simulink model "ES011A_DualEcuIdn"  (R2013b)
settings: Solver=FixedStepDiscrete  SolverMode=SingleTasking  StartTime=0.0  StopTime=1  FixedStep=0.002  RelTol=1e-3
values from neighbouring files (symbols this model uses):
  ECUCOMTIOUTFLT_CNT_U08 = DataDict.Constant    [ES011A_DualEcuIdn_DataDict.m]
  ECUID1_CNT_U08 = DataDict.Constant    [ES011A_DualEcuIdn_DataDict.m]
  ECUID2_CNT_U08 = DataDict.Constant    [ES011A_DualEcuIdn_DataDict.m]
  ECUIDINVLD_CNT_U08 = DataDict.Constant    [ES011A_DualEcuIdn_DataDict.m]
  IDENTCLECUIDNFLT_CNT_U08 = DataDict.Constant    [ES011A_DualEcuIdn_DataDict.m]
  IMCARBN_DUALECUIDNSECDRYECUIDN_CNT_U16 = DataDict.Constant    [ES011A_DualEcuIdn_DataDict.m]
  PRIMECUIDNOTREADFLT_CNT_U08 = DataDict.Constant    [ES011A_DualEcuIdn_DataDict.m]
  PRIMECUINVLDIDFLT_CNT_U08 = DataDict.Constant    [ES011A_DualEcuIdn_DataDict.m]
  SECDRYECUIDNOTREADFLT_CNT_U08 = DataDict.Constant    [ES011A_DualEcuIdn_DataDict.m]
  SECDRYECUIDNREQTIOUTVAL_CNT_U08 = DataDict.Constant    [ES011A_DualEcuIdn_DataDict.m]
  SECDRYECUINVLDIDFLT_CNT_U08 = DataDict.Constant    [ES011A_DualEcuIdn_DataDict.m]
  SECDRYECUREQIDTIOUTFLT_CNT_U08 = DataDict.Constant    [ES011A_DualEcuIdn_DataDict.m]
  VLDECUID_CNT_U08 = DataDict.Constant    [ES011A_DualEcuIdn_DataDict.m]
undefined symbols (not defined in the file or in its folder): NtcNr1, NtcSts1, sigbuilder_block
libraries: simulink x2
(part 2 of 2)

== system ES011A_DualEcuIdn/DualEcuIdn/DualEcuIdnPer1/Evaluation Not Complete/Set Diagnostic 0x0B9/Pass NTC/CopyRight2 ==

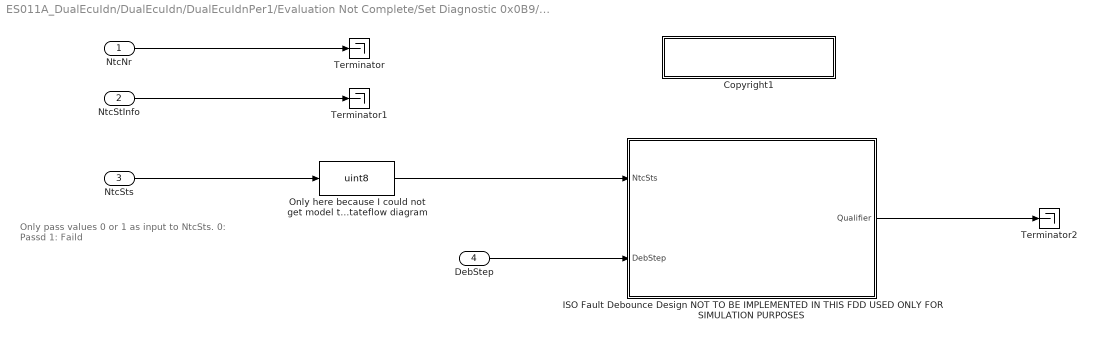
== system ES011A_DualEcuIdn/DualEcuIdn/DualEcuIdnPer1/Evaluation Not Complete/Set Diagnostic 0x0B9/Pass NTC/SetNtcSts ==
  note: Only pass values 0 or 1 as input to NtcSts.
      | 0: Passd
      | 1: Faild
  NtcNr : Inport
  NtcStInfo : Inport  Port=2
  NtcSts : Inport  Port=3  OutDataTypeStr=uint8
  DebStep : Inport  Port=4  OutDataTypeStr=uint16
  Copyright1 : Subsystem  Description=|  mask(Copyright Information){none=on}
      | Copyright info block.                                               
      |                                                                     
      | Place copyright information at the top of every subsystem in design.
      mask prompts: none "No parameters"
      mask help: Place copyright information at the top of every subsystem in design.
      mask Display:
      | NxtrConf = 'Nexteer Confidential';
      | 
      | sys = bdroot; %handle for the current model ("system")
      | first = get_param(sys,'Created');
      | if(isempty(first))
      |     first = datestr(now,'yyyy');
      | else
      |     first = first(end-3:end);  %year is last four digits
      | end
      | 
      | last = get_param(sys,'LastModifiedDate');
      | if isempty(last)
      |     last = datestr(now,'yyyy');
      | else
      |     last = last(end-3:end);
      | end
      | 
      | if strcmp(first,last)
      |     fprintf('%s\nCopyright  %s Nexteer',NxtrConf,first);
      | else
      |     fprintf('%s\n%s%s-%s Nexteer',NxtrConf,char(169),first,last);
      | end
  ISO Fault Debounce Design NOT TO BE IMPLEMENTED IN THIS FDD USED ONLY FOR SIMULATION PURPOSES : Stateflow chart  TreatAsAtomicUnit=on
  Only here because I could not get model to run with enumerations in the stateflow diagram : DataTypeConversion  OutDataTypeStr=uint8
  Terminator : Terminator
  Terminator1 : Terminator
  Terminator2 : Terminator
  wires:
  NtcStInfo/1 -> Terminator1/1
  NtcNr/1 -> Terminator/1
  NtcSts/1 -> Only here because I could not get model to run with enumerations in the stateflow diagram/1
  DebStep/1 -> ISO Fault Debounce Design NOT TO BE IMPLEMENTED IN THIS FDD USED ONLY FOR SIMULATION PURPOSES/2(DebStep)
  ISO Fault Debounce Design NOT TO BE IMPLEMENTED IN THIS FDD USED ONLY FOR SIMULATION PURPOSES/1(Qualifier) -> Terminator2/1
  Only here because I could not get model to run with enumerations in the stateflow diagram/1 -> ISO Fault Debounce Design NOT TO BE IMPLEMENTED IN THIS FDD USED ONLY FOR SIMULATION PURPOSES/1(NtcSts)

== system ES011A_DualEcuIdn/DualEcuIdn/DualEcuIdnPer1/Evaluation Not Complete/Valid Data and E_OK/Different ECU Id/All Good ==
  Action Port : ActionPort  ActionType=else
  CopyRight2 : Subsystem  Description=|  mask(Copyright Information){none=on}
      | Copyright info block.                                               
      |                                                                     
      | Place copyright information at the top of every subsystem in design.
      mask prompts: none "No parameters"
      mask help: Place copyright information at the top of every subsystem in design.
      mask Display:
      | NxtrConf = 'Nexteer Confidential';
      | 
      | sys = bdroot; %handle for the current model ("system")
      | first = get_param(sys,'Created');
      | first = first(end-3:end);  %year is last four digits
      | 
      | last = get_param(sys,'LastModifiedDate');
      | if isempty(last)
      |     last = datestr(now,'yyyy');
      | else
      |     last = last(end-3:end);
      | end
      | 
      | if strcmp(first,last)
      |     fprintf('%s -- Copyright %s Nexteer',NxtrConf,first)
      | else
      |     fprintf('%s -- %s%s- %s Nexteer',NxtrConf,char(169),first,last)
      | end
  Ecu2IdnFail1 : Constant  Value=VLDECUID_CNT_U08
      settings: AttributesFormatString=%<Value>.EngVal = 0
  EcuIdnFltNtc5FPrm : Outport  InitialOutput=0
  wires:
  Ecu2IdnFail1/1 -> EcuIdnFltNtc5FPrm/1

== system ES011A_DualEcuIdn/DualEcuIdn/DualEcuIdnPer1/Evaluation Not Complete/Valid Data and E_OK/Different ECU Id/CopyRight2 ==

== system ES011A_DualEcuIdn/DualEcuIdn/DualEcuIdnPer1/Evaluation Not Complete/Valid Data and E_OK/Different ECU Id/ECU1 ID Not Read ==
  Action Port : ActionPort  ActionType=elseif
  Constant : Constant  Value=PRIMECUIDNOTREADFLT_CNT_U08
      settings: AttributesFormatString=%<Value>.EngVal = 8
  CopyRight2 : Subsystem  Description=|  mask(Copyright Information){none=on}
      | Copyright info block.                                               
      |                                                                     
      | Place copyright information at the top of every subsystem in design.
      mask prompts: none "No parameters"
      mask help: Place copyright information at the top of every subsystem in design.
      mask Display:
      | NxtrConf = 'Nexteer Confidential';
      | 
      | sys = bdroot; %handle for the current model ("system")
      | first = get_param(sys,'Created');
      | first = first(end-3:end);  %year is last four digits
      | 
      | last = get_param(sys,'LastModifiedDate');
      | if isempty(last)
      |     last = datestr(now,'yyyy');
      | else
      |     last = last(end-3:end);
      | end
      | 
      | if strcmp(first,last)
      |     fprintf('%s -- Copyright %s Nexteer',NxtrConf,first)
      | else
      |     fprintf('%s -- %s%s- %s Nexteer',NxtrConf,char(169),first,last)
      | end
  EcuIdnFltNtc5FPrm : Outport  InitialOutput=0
  wires:
  Constant/1 -> EcuIdnFltNtc5FPrm/1

== system ES011A_DualEcuIdn/DualEcuIdn/DualEcuIdnPer1/Evaluation Not Complete/Valid Data and E_OK/Different ECU Id/ECU1 Invalid ID ==
  Action Port : ActionPort  ActionType=then
  Constant : Constant  Value=PRIMECUINVLDIDFLT_CNT_U08
      settings: AttributesFormatString=%<Value>.Engval = 2
  CopyRight2 : Subsystem  Description=|  mask(Copyright Information){none=on}
      | Copyright info block.                                               
      |                                                                     
      | Place copyright information at the top of every subsystem in design.
      mask prompts: none "No parameters"
      mask help: Place copyright information at the top of every subsystem in design.
      mask Display:
      | NxtrConf = 'Nexteer Confidential';
      | 
      | sys = bdroot; %handle for the current model ("system")
      | first = get_param(sys,'Created');
      | first = first(end-3:end);  %year is last four digits
      | 
      | last = get_param(sys,'LastModifiedDate');
      | if isempty(last)
      |     last = datestr(now,'yyyy');
      | else
      |     last = last(end-3:end);
      | end
      | 
      | if strcmp(first,last)
      |     fprintf('%s -- Copyright %s Nexteer',NxtrConf,first)
      | else
      |     fprintf('%s -- %s%s- %s Nexteer',NxtrConf,char(169),first,last)
      | end
  EcuIdnFltNtc5FPrm : Outport  InitialOutput=0
  wires:
  Constant/1 -> EcuIdnFltNtc5FPrm/1

== system ES011A_DualEcuIdn/DualEcuIdn/DualEcuIdnPer1/Evaluation Not Complete/Valid Data and E_OK/Different ECU Id/ECU2 ID Not Read ==
  Action Port : ActionPort  ActionType=elseif
  Constant : Constant  Value=SECDRYECUIDNOTREADFLT_CNT_U08
      settings: AttributesFormatString=%<Value>.EngVal = 16
  CopyRight2 : Subsystem  Description=|  mask(Copyright Information){none=on}
      | Copyright info block.                                               
      |                                                                     
      | Place copyright information at the top of every subsystem in design.
      mask prompts: none "No parameters"
      mask help: Place copyright information at the top of every subsystem in design.
      mask Display:
      | NxtrConf = 'Nexteer Confidential';
      | 
      | sys = bdroot; %handle for the current model ("system")
      | first = get_param(sys,'Created');
      | first = first(end-3:end);  %year is last four digits
      | 
      | last = get_param(sys,'LastModifiedDate');
      | if isempty(last)
      |     last = datestr(now,'yyyy');
      | else
      |     last = last(end-3:end);
      | end
      | 
      | if strcmp(first,last)
      |     fprintf('%s -- Copyright %s Nexteer',NxtrConf,first)
      | else
      |     fprintf('%s -- %s%s- %s Nexteer',NxtrConf,char(169),first,last)
      | end
  EcuIdnFltNtc5FPrm : Outport  InitialOutput=0
  wires:
  Constant/1 -> EcuIdnFltNtc5FPrm/1

== system ES011A_DualEcuIdn/DualEcuIdn/DualEcuIdnPer1/Evaluation Not Complete/Valid Data and E_OK/Different ECU Id/ECU2 Invalid ID ==
  Action Port : ActionPort  ActionType=elseif
  Constant : Constant  Value=SECDRYECUINVLDIDFLT_CNT_U08
      settings: AttributesFormatString=%<Value>.EngVal = 4
  CopyRight2 : Subsystem  Description=|  mask(Copyright Information){none=on}
      | Copyright info block.                                               
      |                                                                     
      | Place copyright information at the top of every subsystem in design.
      mask prompts: none "No parameters"
      mask help: Place copyright information at the top of every subsystem in design.
      mask Display:
      | NxtrConf = 'Nexteer Confidential';
      | 
      | sys = bdroot; %handle for the current model ("system")
      | first = get_param(sys,'Created');
      | first = first(end-3:end);  %year is last four digits
      | 
      | last = get_param(sys,'LastModifiedDate');
      | if isempty(last)
      |     last = datestr(now,'yyyy');
      | else
      |     last = last(end-3:end);
      | end
      | 
      | if strcmp(first,last)
      |     fprintf('%s -- Copyright %s Nexteer',NxtrConf,first)
      | else
      |     fprintf('%s -- %s%s- %s Nexteer',NxtrConf,char(169),first,last)
      | end
  EcuIdnFltNtc5FPrm : Outport  InitialOutput=0
  wires:
  Constant/1 -> EcuIdnFltNtc5FPrm/1

== system ES011A_DualEcuIdn/DualEcuIdn/DualEcuIdnPer1/Evaluation Not Complete/Valid Data and E_OK/Same ECU Id/CopyRight2 ==

== system ES011A_DualEcuIdn/DualEcuIdn/DualEcuIdnPer1/Evaluation Not Complete/Set Diagnostic 0x0B9/Fail NTC/SetNtcSts/Copyright1 ==

== system ES011A_DualEcuIdn/DualEcuIdn/DualEcuIdnPer1/Evaluation Not Complete/Set Diagnostic 0x0B9/Pass NTC/SetNtcSts/Copyright1 ==

== system ES011A_DualEcuIdn/DualEcuIdn/DualEcuIdnPer1/Evaluation Not Complete/Valid Data and E_OK/Different ECU Id/All Good/CopyRight2 ==

== system ES011A_DualEcuIdn/DualEcuIdn/DualEcuIdnPer1/Evaluation Not Complete/Valid Data and E_OK/Different ECU Id/ECU1 ID Not Read/CopyRight2 ==

== system ES011A_DualEcuIdn/DualEcuIdn/DualEcuIdnPer1/Evaluation Not Complete/Valid Data and E_OK/Different ECU Id/ECU1 Invalid ID/CopyRight2 ==

== system ES011A_DualEcuIdn/DualEcuIdn/DualEcuIdnPer1/Evaluation Not Complete/Valid Data and E_OK/Different ECU Id/ECU2 ID Not Read/CopyRight2 ==

== system ES011A_DualEcuIdn/DualEcuIdn/DualEcuIdnPer1/Evaluation Not Complete/Valid Data and E_OK/Different ECU Id/ECU2 Invalid ID/CopyRight2 ==

== stateflow chart ES011A_DualEcuIdn/DualEcuIdn/DualEcuIdnPer1/Evaluation Not Complete/Set Diagnostic 0x0B9/Fail NTC/SetNtcSts/ISO Fault Debounce Design NOT TO BE IMPLEMENTED IN THIS FDD USED ONLY FOR SIMULATION PURPOSES ==
  note: NTCSTS_PASSD           (0)
      | NTCSTS_FAILD             (1)
      | NTCSTS_PREPASSD   (2)
      | NTCSTS_PREFAILD     (3)
      |
      | SIGQLFR_NORES        (0)
      | SIGQLFR_PASSD         (1)
      | SIGQLFR_FAILD           (2)
  (default) -> (junction 221)
  (junction 221) -> (junction 212) [order 2] : [NtcSts == 0]
      | {
      | DebCntr = -32768;
      | Qualifier=1;
      | }
  (junction 221) -> (junction 212) [order 1] : [NtcSts == 1]
      | {
      | DebCntr = 32767;
      | Qualifier =2;
      |  }
  (junction 212) -> (junction 159)
  data: NtcSts input uint8; Qualifier output uint8 =0; DebStep input uint16; DebCntr local int16

== stateflow chart ES011A_DualEcuIdn/DualEcuIdn/DualEcuIdnPer1/Evaluation Not Complete/Set Diagnostic 0x0B9/Pass NTC/SetNtcSts/ISO Fault Debounce Design NOT TO BE IMPLEMENTED IN THIS FDD USED ONLY FOR SIMULATION PURPOSES ==
  note: NTCSTS_PASSD           (0)
      | NTCSTS_FAILD             (1)
      | NTCSTS_PREPASSD   (2)
      | NTCSTS_PREFAILD     (3)
      |
      | SIGQLFR_NORES        (0)
      | SIGQLFR_PASSD         (1)
      | SIGQLFR_FAILD           (2)
  (default) -> (junction 221)
  (junction 221) -> (junction 212) [order 2] : [NtcSts == 0]
      | {
      | DebCntr = -32768;
      | Qualifier=1;
      | }
  (junction 221) -> (junction 212) [order 1] : [NtcSts == 1]
      | {
      | DebCntr = 32767;
      | Qualifier =2;
      |  }
  (junction 212) -> (junction 159)
  data: NtcSts input uint8; Qualifier output uint8 =0; DebStep input uint16; DebCntr local int16
